simulink subsystem "Equations_of_Motion"  (R2023b)
settings: Solver=VariableStepAuto  StartTime=0.0  StopTime=10.0  RelTol=1e-3
undefined symbols (not defined in the file): CNT_g, CNT_m, Iyy, TrimPoint
settings Model: Creator=NicolasS  LastModifiedBy=rouve
settings SolverCC: AlgebraicLoopSolver=TrustRegion
settings DebuggingCC: UnconnectedInputMsg=warning  UnconnectedOutputMsg=warning  UnconnectedLineMsg=warning
settings ModelReferenceCC: EnableRefExpFcnMdlSchedulingChecks=on
settings RTWCC: DLArmComputeVersion=19.05

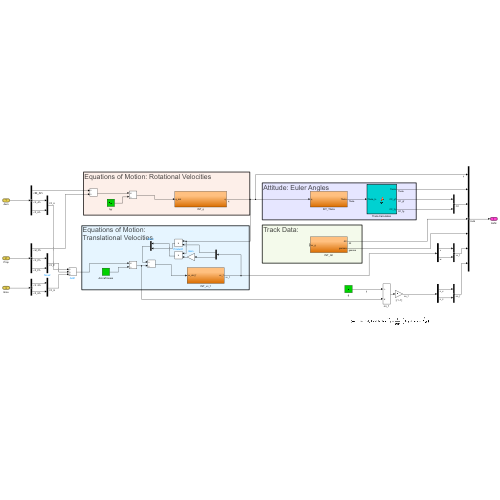
[thumbnail: Simulink's stored preview of the top-level diagram]
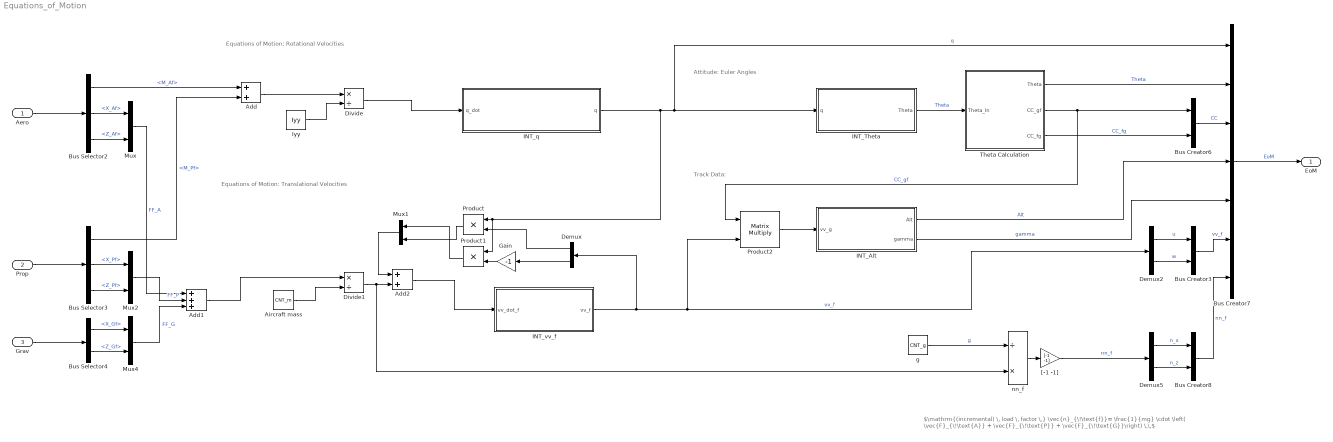
== system Equations_of_Motion ==
  note: Attitude: Euler Angles
  note: $\mathrm{(incremental) \, load \, factor \,} \vec{n}_{\!\text{f}}= \frac{1}{mg} \cdot \left( \vec{F}_{\!\text{A}} + \vec{F}_{\!\text{P}} + \vec{F}_{\!\text{G}}\right) \,\,$
  note: Track Data:
  note: Equations of Motion: Rotational Velocities
  note: Equations of Motion:
      | Translational Velocities
  Aero : Inport  OutDataTypeStr=Bus: Aero
  Prop : Inport  Port=2  OutDataTypeStr=Bus: Prop
  Grav : Inport  Port=3  OutDataTypeStr=Bus: Grav
  Add : Sum
  Add1 : Sum  Inputs=+++
  Add2 : Sum
  Aircraft mass : Constant  Value=CNT_m  SampleTime=-1
  Bus Creator3 : BusCreator  Inputs=2  OutDataTypeStr=Bus: vv_f
  Bus Creator6 : BusCreator  Inputs=2  OutDataTypeStr=Bus: CC
  Bus Creator7 : BusCreator  Inputs=7  OutDataTypeStr=Bus: EoM
  Bus Creator8 : BusCreator  Inputs=2  OutDataTypeStr=Bus: nn_f
  Bus Selector2 : BusSelector  OutputSignals=M_Af,X_Af,Z_Af
  Bus Selector3 : BusSelector  OutputSignals=M_Pf,X_Pf,Z_Pf
  Bus Selector4 : BusSelector  OutputSignals=X_Gf,Z_Gf
  Demux : Demux  Outputs=2
  Demux2 : Demux  Outputs=2
  Demux5 : Demux  Outputs=2
  Divide : Product  Inputs=*/
  Divide1 : Product  Inputs=*/
  Gain : Gain  Gain=-1
  INT_Alt : Subsystem
  INT_Theta : Subsystem
  INT_q : Subsystem
  INT_vv_f : Subsystem
  Iyy : Constant  Value=Iyy  SampleTime=-1
  Mux{,1..2,4} (4 alike) : Mux  Inputs=2
  Product : Product
  Product1 : Product
  Product2 : Product  Multiplication=Matrix(*)
  Theta Calculation : MATLAB Function  TreatAsAtomicUnit=on
  "[-1 -1]" : Gain  Gain=[-1 -1]
  g : Constant  Value=CNT_g  SampleTime=-1
  "nn_f " : Product  Inputs=/*  RndMeth=Zero
  EoM : Outport  OutDataTypeStr=Bus: EoM
  wires:
  Bus Selector3/2 -> Mux2/1  "<X_Pf>"
  Theta Calculation/2(CC_gf) -> Bus Creator6/1, Product2/1  "CC_gf"
  Bus Creator8/1 -> Bus Creator7/7  "nn_f"
  "nn_f "/1 -> "[-1 -1]"/1
  Bus Selector4/1 -> Mux4/1  "<X_Gf>"
  Bus Selector3/1 -> Add/2  "<M_Pf>"
  INT_Theta/1(Theta) -> Theta Calculation/1(Theta_In)  "Theta"
  Bus Creator3/1 -> Bus Creator7/6  "vv_f"
  INT_Alt/2(gamma) -> Bus Creator7/5  "gamma"
  Bus Creator6/1 -> Bus Creator7/3  "CC"
  Theta Calculation/1(Theta) -> Bus Creator7/2  "Theta"
  Bus Selector2/3 -> Mux/2  "<Z_Af>"
  Aircraft mass/1 -> Divide1/2
  Demux5/1 -> Bus Creator8/1  "n_x"
  INT_q/1(q) -> Product1/1, Product/1, Bus Creator7/1, INT_Theta/1(q)  "q"
  Bus Selector4/2 -> Mux4/2  "<Z_Gf>"
  g/1 -> "nn_f "/1  "g"
  Bus Selector2/2 -> Mux/1  "<X_Af>"
  Aero/1 -> Bus Selector2/1
  Bus Selector2/1 -> Add/1  "<M_Af>"
  Demux5/2 -> Bus Creator8/2  "n_z"
  Iyy/1 -> Divide/2
  Grav/1 -> Bus Selector4/1
  Prop/1 -> Bus Selector3/1
  INT_vv_f/1(vv_f) -> Demux/1, Demux2/1, Product2/2  "vv_f"
  Demux2/2 -> Bus Creator3/2  "w"
  Bus Selector3/3 -> Mux2/2  "<Z_Pf>"
  Demux2/1 -> Bus Creator3/1  "u"
  Mux/1 -> Add1/1  "FF_A"
  "[-1 -1]"/1 -> Demux5/1  "nn_f"
  INT_Alt/1(Alt) -> Bus Creator7/4  "Alt"
  Theta Calculation/3(CC_fg) -> Bus Creator6/2  "CC_fg"
  Add/1 -> Divide/1
  Divide/1 -> INT_q/1(q_dot)
  Mux2/1 -> Add1/2  "FF_P"
  Mux4/1 -> Add1/3  "FF_G"
  Demux/1 -> Product/2
  Demux/2 -> Gain/1
  Gain/1 -> Product1/2
  Product1/1 -> Mux1/1
  Product/1 -> Mux1/2
  Mux1/1 -> Add2/1
  Divide1/1 -> "nn_f "/2, Add2/2
  Add2/1 -> INT_vv_f/1(vv_dot_f)
  Add1/1 -> Divide1/1
  Product2/1 -> INT_Alt/1(vv_g)
  Bus Creator7/1 -> EoM/1  "EoM"

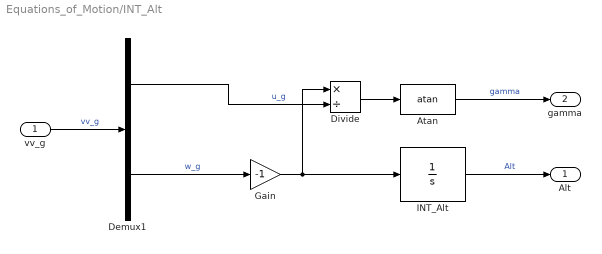
== system Equations_of_Motion/INT_Alt ==
  vv_g : Inport
  Atan : Trigonometry  Operator=atan
  Demux1 : Demux  Outputs=2
  Divide : Product  Inputs=*/
  Gain : Gain  Gain=-1
  INT_Alt : Integrator  InitialCondition=TrimPoint.States.Altbar  ContinuousStateAttributes='Alt'
  Alt : Outport
  gamma : Outport  Port=2
  wires:
  Divide/1 -> Atan/1
  Gain/1 -> Divide/1, INT_Alt/1
  INT_Alt/1 -> Alt/1  "Alt"
  vv_g/1 -> Demux1/1  "vv_g"
  Demux1/2 -> Gain/1  "w_g"
  Demux1/1 -> Divide/2  "u_g"
  Atan/1 -> gamma/1  "gamma"

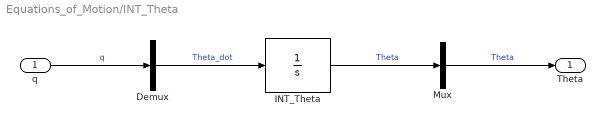
== system Equations_of_Motion/INT_Theta ==
  q : Inport
  Demux : Demux  Outputs=1
  INT_Theta : Integrator  InitialCondition=TrimPoint.States.Thetabar  ContinuousStateAttributes='Theta'
  Mux : Mux  Inputs=1
  Theta : Outport
  wires:
  Mux/1 -> Theta/1  "Theta"
  INT_Theta/1 -> Mux/1  "Theta"
  Demux/1 -> INT_Theta/1  "Theta_dot"
  q/1 -> Demux/1  "q"

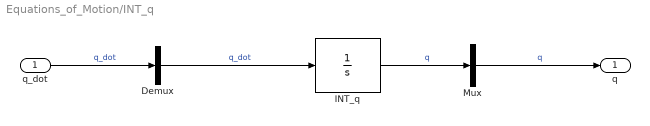
== system Equations_of_Motion/INT_q ==
  q_dot : Inport
  Demux : Demux  Outputs=1
  INT_q : Integrator  InitialCondition=TrimPoint.States.qbar  ContinuousStateAttributes='q'
  Mux : Mux  Inputs=1
  q : Outport
  wires:
  Mux/1 -> q/1  "q"
  INT_q/1 -> Mux/1  "q"
  Demux/1 -> INT_q/1  "q_dot"
  q_dot/1 -> Demux/1  "q_dot"

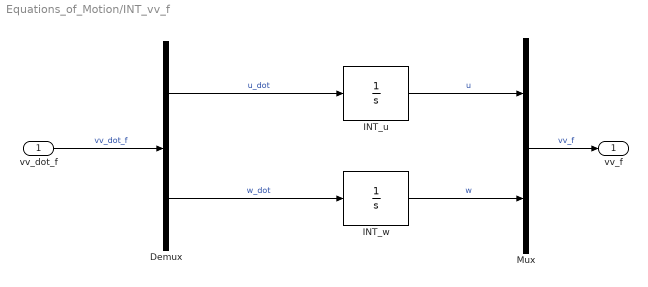
== system Equations_of_Motion/INT_vv_f ==
  vv_dot_f : Inport
  Demux : Demux  Outputs=2
  INT_u : Integrator  InitialCondition=TrimPoint.States.ubar  ContinuousStateAttributes='u'
  INT_w : Integrator  InitialCondition=TrimPoint.States.wbar  ContinuousStateAttributes='w'
  Mux : Mux  Inputs=2
  vv_f : Outport
  wires:
  vv_dot_f/1 -> Demux/1  "vv_dot_f"
  Demux/1 -> INT_u/1  "u_dot"
  Demux/2 -> INT_w/1  "w_dot"
  INT_u/1 -> Mux/1  "u"
  INT_w/1 -> Mux/2  "w"
  Mux/1 -> vv_f/1  "vv_f"

== matlab function Equations_of_Motion/Theta Calculation ==
  data: Theta output size=1; CC_gf output size=[2 2]; CC_fg output size=[2 2]; Theta_In input size=1
function [Theta,CC_gf,CC_fg] = fcn(Theta_In)

Theta = mod(Theta_In+pi,2*pi)-pi; % pi bound

CC_fg = [cos(Theta), -sin(Theta); sin(Theta), cos(Theta)];
     
CC_gf = [cos(Theta), sin(Theta); -sin(Theta), cos(Theta)];
